simulink model "SIMULINK_EX_IV"  (R2021a)
settings: Solver=VariableStepAuto  StartTime=0.0  StopTime=10.0  RelTol=1e-3
settings Model: Creator=GHOST  LastModifiedBy=GHOST

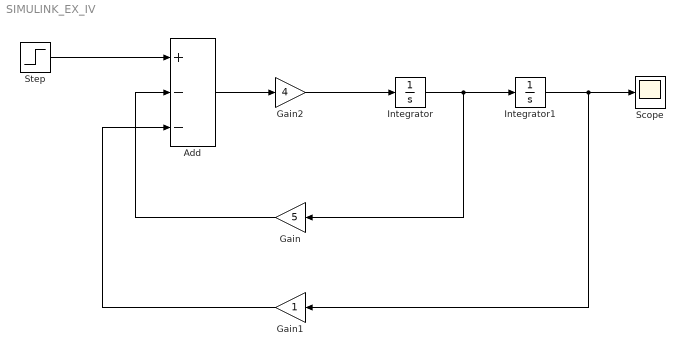
== system SIMULINK_EX_IV ==
  Add : Sum  Inputs=+--
  Gain : Gain  Gain=5
  Gain1 : Gain
  Gain2 : Gain  Gain=4
  Integrator : Integrator
  Integrator1 : Integrator
  Scope : Scope
  Step : Step  Before=3  After=2  SampleTime=0
  wires:
  Integrator1/1 -> Gain1/1, Scope/1
  Integrator/1 -> Gain/1, Integrator1/1
  Gain/1 -> Add/2
  Add/1 -> Gain2/1
  Gain2/1 -> Integrator/1
  Gain1/1 -> Add/3
  Step/1 -> Add/1
